simulink model "airbrakes"  (R2025b)
settings: Solver=VariableStepAuto  StartTime=0.0  StopTime=10.0  RelTol=1e-3
values from neighbouring files (symbols this model uses):
  baro_bias_initial = 1.0    (= 1)    [init_airbrake_model.m]
  baro_sigma_h = 0.5    [init_airbrake_model.m]
  burnout_time = motor_time(end)    [init_airbrake_model.m]
  Cd_body_bp = [0.45 0.45 0.43 0.42 0.44 0.50 0.65 0.75 0.62 0.52 0.48]    [init_airbrake_model.m]
  DeltaCd_ab_table = [ ... (first row only)    [init_airbrake_model.m]
  deploy_bp = [0 0.25 0.50 0.75 1.00]    [init_airbrake_model.m]
  deploy_rate_down = 6.67    [init_airbrake_model.m]
  deploy_rate_up = 6.67    [init_airbrake_model.m]
  g0 = 9.80665    [init_airbrake_model.m]
  imu_accel_range_g = 16    [init_airbrake_model.m]
  imu_bias_initial = 0.05    [init_airbrake_model.m]
  imu_delay = 0.005    [init_airbrake_model.m]
  imu_sigma_a = 0.15    [init_airbrake_model.m]
  Mach_ab_bp = Mach_bp    [init_airbrake_model.m]
  Mach_bp = [0 0.1 0.3 0.5 0.7 0.85 0.95 1.05 1.2 1.5 2.0]    [init_airbrake_model.m]
  mass_curve = linspace(m0, m_dry, numel(mass_time))    [init_airbrake_model.m]
  mass_time = motor_time    [init_airbrake_model.m]
  motor_thrust = [0 1200 2500 3300 3400 3200 2800 1900 700 100 0]    [init_airbrake_model.m]
  motor_time = [0 0.05 0.10 0.50 1.00 1.50 2.00 2.50 3.00 3.20 3.30]    [init_airbrake_model.m]
  Ts_baro = 0.02    [init_airbrake_model.m]
  Ts_imu = 0.005    [init_airbrake_model.m]
undefined symbols (not defined in the file or in its folder): bldc_tau
libraries: simulink x4
settings Model: Creator=parsa  LastModifiedBy=parsa

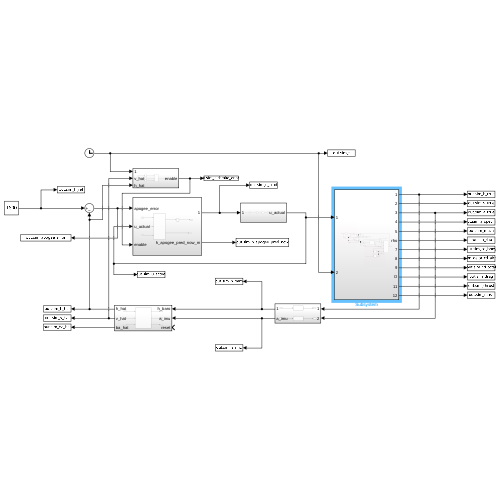
[thumbnail: Simulink's stored preview of the top-level diagram]
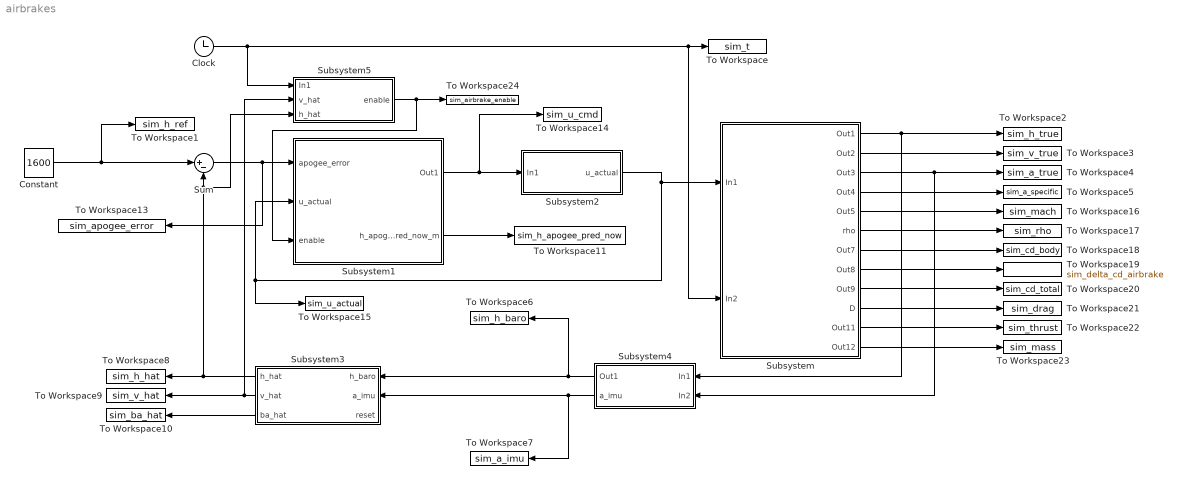
== system airbrakes ==
  Clock : Clock
  Constant : Constant  Value=1600
  Subsystem : Subsystem
  Subsystem1 : Subsystem
  Subsystem2 : Subsystem
  Subsystem3 : Subsystem
  Subsystem4 : Subsystem
  Subsystem5 : Subsystem
  Sum : Sum  Inputs=|+-
  To Workspace : ToWorkspace  VariableName=sim_t  SaveFormat=Timeseries  SampleTime=-1
  To Workspace1 : ToWorkspace  VariableName=sim_h_ref  SaveFormat=Timeseries  SampleTime=-1
  To Workspace10 : ToWorkspace  VariableName=sim_ba_hat  SaveFormat=Timeseries  SampleTime=-1
  To Workspace11 : ToWorkspace  VariableName=sim_h_apogee_pred_now  SaveFormat=Timeseries  SampleTime=-1
  To Workspace13 : ToWorkspace  VariableName=sim_apogee_error  SaveFormat=Timeseries  SampleTime=-1
  To Workspace14 : ToWorkspace  VariableName=sim_u_cmd  SaveFormat=Timeseries  SampleTime=-1
  To Workspace15 : ToWorkspace  VariableName=sim_u_actual  SaveFormat=Timeseries  SampleTime=-1
  To Workspace16 : ToWorkspace  VariableName=sim_mach  SaveFormat=Timeseries  SampleTime=-1
  To Workspace17 : ToWorkspace  VariableName=sim_rho  SaveFormat=Timeseries  SampleTime=-1
  To Workspace18 : ToWorkspace  VariableName=sim_cd_body  SaveFormat=Timeseries  SampleTime=-1
  To Workspace19 : ToWorkspace  VariableName=sim_delta_cd_airbrake  SaveFormat=Timeseries  SampleTime=-1
  To Workspace2 : ToWorkspace  VariableName=sim_h_true  SaveFormat=Timeseries  SampleTime=-1
  To Workspace20 : ToWorkspace  VariableName=sim_cd_total  SaveFormat=Timeseries  SampleTime=-1
  To Workspace21 : ToWorkspace  VariableName=sim_drag  SaveFormat=Timeseries  SampleTime=-1
  To Workspace22 : ToWorkspace  VariableName=sim_thrust  SaveFormat=Timeseries  SampleTime=-1
  To Workspace23 : ToWorkspace  VariableName=sim_mass  SaveFormat=Timeseries  SampleTime=-1
  To Workspace24 : ToWorkspace  VariableName=sim_airbrake_enable  SaveFormat=Timeseries  SampleTime=-1
  To Workspace3 : ToWorkspace  VariableName=sim_v_true  SaveFormat=Timeseries  SampleTime=-1
  To Workspace4 : ToWorkspace  VariableName=sim_a_true  SaveFormat=Timeseries  SampleTime=-1
  To Workspace5 : ToWorkspace  VariableName=sim_a_specific  SaveFormat=Timeseries  SampleTime=-1
  To Workspace6 : ToWorkspace  VariableName=sim_h_baro  SaveFormat=Timeseries  SampleTime=-1
  To Workspace7 : ToWorkspace  VariableName=sim_a_imu  SaveFormat=Timeseries  SampleTime=-1
  To Workspace8 : ToWorkspace  VariableName=sim_h_hat  SaveFormat=Timeseries  SampleTime=-1
  To Workspace9 : ToWorkspace  VariableName=sim_v_hat  SaveFormat=Timeseries  SampleTime=-1
  wires:
  Subsystem4/1(Out1) -> To Workspace6/1, Subsystem3/1(h_baro)
  Subsystem1/1(Out1) -> To Workspace14/1, Subsystem2/1(In1)
  Subsystem3/1(h_hat) -> Subsystem5/3(h_hat), Sum/2, To Workspace8/1
  Constant/1 -> To Workspace1/1, Sum/1
  Subsystem2/1(u_actual) -> To Workspace15/1, Subsystem1/2(u_actual), Subsystem/1(In1)
  Subsystem4/2(a_imu) -> To Workspace7/1, Subsystem3/2(a_imu)
  Clock/1 -> Subsystem5/1(In1), Subsystem/2(In2), To Workspace/1
  Subsystem3/2(v_hat) -> To Workspace9/1, Subsystem5/2(v_hat)
  Sum/1 -> To Workspace13/1, Subsystem1/1(apogee_error)
  Subsystem5/1(enable) -> To Workspace24/1, Subsystem1/3(enable)
  Subsystem3/3(ba_hat) -> To Workspace10/1
  Subsystem1/2(h_apogee_pred_now_m) -> To Workspace11/1
  Subsystem/1(Out1) -> Subsystem4/1(In1), To Workspace2/1
  Subsystem/2(Out2) -> To Workspace3/1
  Subsystem/3(Out3) -> Subsystem4/2(In2), To Workspace4/1
  Subsystem/4(Out4) -> To Workspace5/1
  Subsystem/5(Out5) -> To Workspace16/1
  Subsystem/6(rho) -> To Workspace17/1
  Subsystem/7(Out7) -> To Workspace18/1
  Subsystem/8(Out8) -> To Workspace19/1
  Subsystem/9(Out9) -> To Workspace20/1
  Subsystem/10(D) -> To Workspace21/1
  Subsystem/11(Out11) -> To Workspace22/1
  Subsystem/12(Out12) -> To Workspace23/1

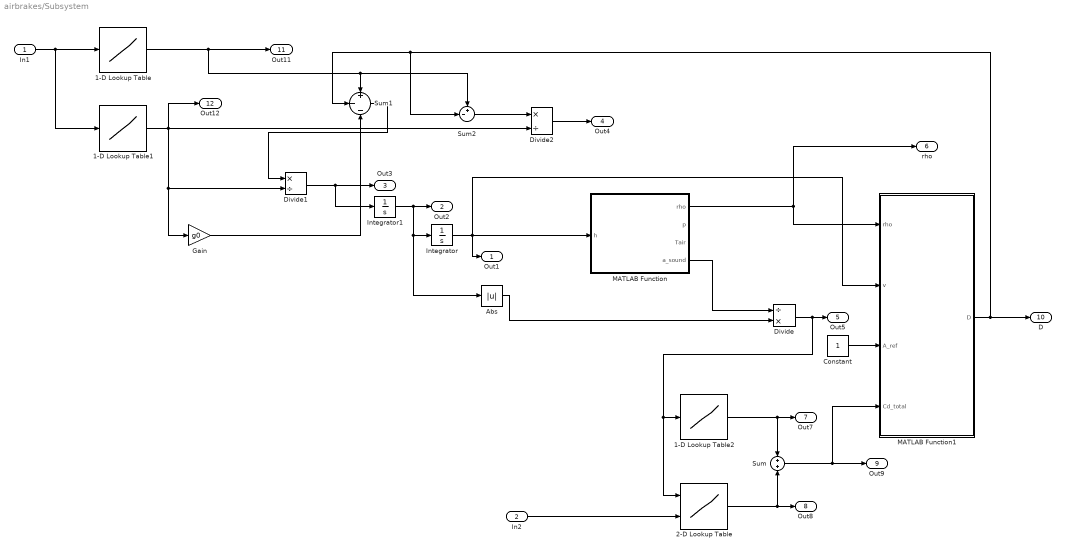
== system airbrakes/Subsystem ==
  In1 : Inport
  In2 : Inport  Port=2
  1-D Lookup Table : Lookup_n-D  NumberOfTableDimensions=1  BreakpointsForDimension1=motor_thrust  Table=motor_time  InternalRulePriority=Speed  RndMeth=Simplest
  1-D Lookup Table1 : Lookup_n-D  NumberOfTableDimensions=1  BreakpointsForDimension1=mass_time  Table=mass_curve  InternalRulePriority=Speed  RndMeth=Simplest
  1-D Lookup Table2 : Lookup_n-D  NumberOfTableDimensions=1  BreakpointsForDimension1=Mach_bp  Table=Cd_body_bp  InternalRulePriority=Speed  RndMeth=Simplest
  2-D Lookup Table : Lookup_n-D  BreakpointsForDimension1=deploy_bp  BreakpointsForDimension2=Mach_ab_bp  Table=DeltaCd_ab_table  InternalRulePriority=Speed  RndMeth=Simplest
      settings: InputPortMap=u0,u1
  Abs : Abs  SaturateOnIntegerOverflow=off
  Constant : Constant
  Divide : Product  Inputs=/*
  Divide1 : Product  Inputs=*/
  Divide2 : Product  Inputs=*/
  Gain : Gain  Gain=g0
  Integrator : Integrator
  Integrator1 : Integrator
  MATLAB Function : MATLAB Function  TreatAsAtomicUnit=on
  MATLAB Function1 : MATLAB Function  TreatAsAtomicUnit=on
  Sum : Sum  Inputs=+|+
  Sum1 : Sum  Inputs=+|-|-
  Sum2 : Sum  Inputs=+-|
  Out1 : Outport
  Out2 : Outport  Port=2
  Out3 : Outport  Port=3
  Out4 : Outport  Port=4
  Out5 : Outport  Port=5
  rho : Outport  Port=6
  Out7 : Outport  Port=7
  Out8 : Outport  Port=8
  Out9 : Outport  Port=9
  D : Outport  Port=10
  Out11 : Outport  Port=11
  Out12 : Outport  Port=12
  wires:
  In1/1 -> 1-D Lookup Table1/1, 1-D Lookup Table/1
  1-D Lookup Table/1 -> Sum2/1, Sum1/1, Out11/1
  1-D Lookup Table1/1 -> Out12/1, Divide2/2, Gain/1, Divide1/2
  Sum1/1 -> Divide1/1
  Divide1/1 -> Integrator1/1, Out3/1
  Integrator1/1 -> Out2/1, Abs/1, Integrator/1
  Integrator/1 -> Out1/1, MATLAB Function/1(h), MATLAB Function1/2(v)
  MATLAB Function/1(rho) -> MATLAB Function1/1(rho), rho/1
  MATLAB Function/4(a_sound) -> Divide/1
  Abs/1 -> Divide/2
  Divide/1 -> 2-D Lookup Table/1, 1-D Lookup Table2/1, Out5/1
  In2/1 -> 2-D Lookup Table/2
  1-D Lookup Table2/1 -> Out7/1, Sum/1
  2-D Lookup Table/1 -> Out8/1, Sum/2
  Sum/1 -> Out9/1, MATLAB Function1/4(Cd_total)
  Gain/1 -> Sum1/3
  MATLAB Function1/1(D) -> D/1, Sum2/2, Sum1/2
  Constant/1 -> MATLAB Function1/3(A_ref)
  Sum2/1 -> Divide2/1
  Divide2/1 -> Out4/1

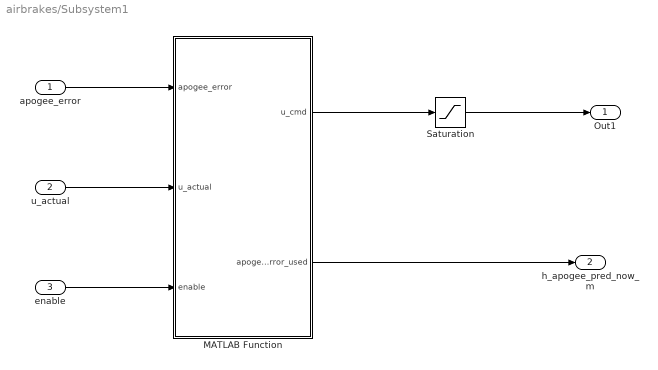
== system airbrakes/Subsystem1 ==
  apogee_error : Inport
  u_actual : Inport  Port=2
  enable : Inport  Port=3
  MATLAB Function : MATLAB Function  TreatAsAtomicUnit=on
  Saturation : Saturate  UpperLimit=1  LowerLimit=0
  Out1 : Outport
  h_apogee_pred_now_m : Outport  Port=2
  wires:
  MATLAB Function/1(u_cmd) -> Saturation/1
  Saturation/1 -> Out1/1
  MATLAB Function/2(apogee_error_used) -> h_apogee_pred_now_m/1
  enable/1 -> MATLAB Function/3(enable)
  u_actual/1 -> MATLAB Function/2(u_actual)
  apogee_error/1 -> MATLAB Function/1(apogee_error)

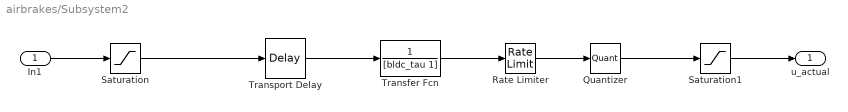
== system airbrakes/Subsystem2 ==
  In1 : Inport
  Quantizer : Quantizer  QuantizationInterval=bldc_quant_step
  Rate Limiter : RateLimiter  RisingSlewLimit=deploy_rate_up  FallingSlewLimit=-deploy_rate_down  SampleTimeMode=inherited
  Saturation : Saturate  UpperLimit=1  LowerLimit=0
  Saturation1 : Saturate  UpperLimit=1  LowerLimit=0
  Transfer Fcn : TransferFcn  Denominator=[bldc_tau 1]
  Transport Delay : TransportDelay
  u_actual : Outport
  wires:
  In1/1 -> Saturation/1
  Saturation/1 -> Transport Delay/1
  Transport Delay/1 -> Transfer Fcn/1
  Transfer Fcn/1 -> Rate Limiter/1
  Rate Limiter/1 -> Quantizer/1
  Quantizer/1 -> Saturation1/1
  Saturation1/1 -> u_actual/1

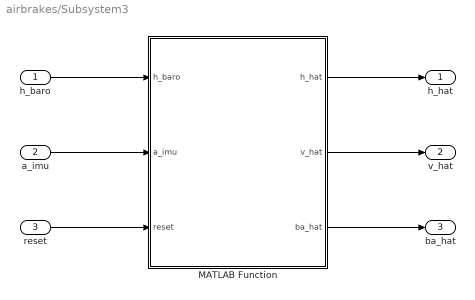
== system airbrakes/Subsystem3 ==
  h_baro : Inport
  a_imu : Inport  Port=2
  reset : Inport  Port=3
  MATLAB Function : MATLAB Function  TreatAsAtomicUnit=on
  h_hat : Outport
  v_hat : Outport  Port=2
  ba_hat : Outport  Port=3
  wires:
  reset/1 -> MATLAB Function/3(reset)
  a_imu/1 -> MATLAB Function/2(a_imu)
  h_baro/1 -> MATLAB Function/1(h_baro)
  MATLAB Function/1(h_hat) -> h_hat/1
  MATLAB Function/2(v_hat) -> v_hat/1
  MATLAB Function/3(ba_hat) -> ba_hat/1

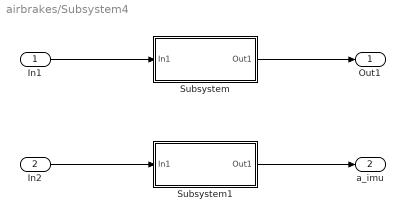
== system airbrakes/Subsystem4 ==
  In1 : Inport
  In2 : Inport  Port=2
  Subsystem : Subsystem
  Subsystem1 : Subsystem
  Out1 : Outport
  a_imu : Outport  Port=2
  wires:
  In2/1 -> Subsystem1/1(In1)
  Subsystem1/1(Out1) -> a_imu/1
  Subsystem/1(Out1) -> Out1/1
  In1/1 -> Subsystem/1(In1)

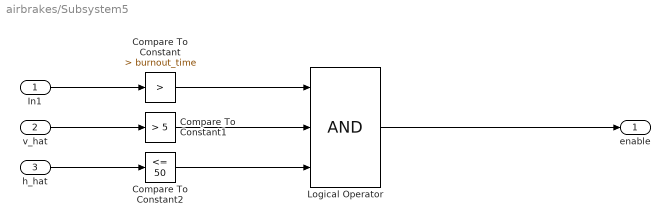
== system airbrakes/Subsystem5 ==
  In1 : Inport
  v_hat : Inport  Port=2
  h_hat : Inport  Port=3
  Compare To Constant : simulink/Logic and Bit Operations/Compare To Constant  relop=>  const=burnout_time  OutDataTypeStr=boolean
  Compare To Constant1 : simulink/Logic and Bit Operations/Compare To Constant  relop=>  const=5  OutDataTypeStr=boolean
  Compare To Constant2 : simulink/Logic and Bit Operations/Compare To Constant  relop=<=  const=50  OutDataTypeStr=boolean
  Logical Operator : Logic  Inputs=3  AllPortsSameDT=off  OutDataTypeStr=boolean
  enable : Outport
  wires:
  In1/1 -> Compare To Constant/1
  Compare To Constant/1 -> Logical Operator/1
  v_hat/1 -> Compare To Constant1/1
  h_hat/1 -> Compare To Constant2/1
  Compare To Constant1/1 -> Logical Operator/2
  Compare To Constant2/1 -> Logical Operator/3
  Logical Operator/1 -> enable/1

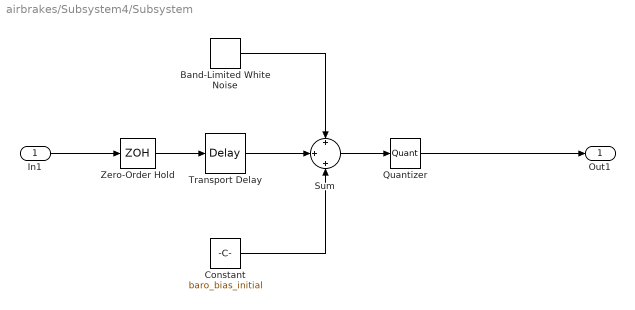
== system airbrakes/Subsystem4/Subsystem ==
  In1 : Inport
  Band-Limited White Noise : simulink/Sources/Band-Limited White Noise  Cov=[baro_sigma_h^2 * Ts_baro]  Ts=Ts_baro  seed=[23341]
  Constant : Constant  Value=baro_bias_initial
  Quantizer : Quantizer
  Sum : Sum  Inputs=+|+|+
  Transport Delay : TransportDelay
  Zero-Order Hold : ZeroOrderHold  SampleTime=-1
  Out1 : Outport
  wires:
  In1/1 -> Zero-Order Hold/1
  Zero-Order Hold/1 -> Transport Delay/1
  Band-Limited White Noise/1 -> Sum/1
  Transport Delay/1 -> Sum/2
  Constant/1 -> Sum/3
  Sum/1 -> Quantizer/1
  Quantizer/1 -> Out1/1

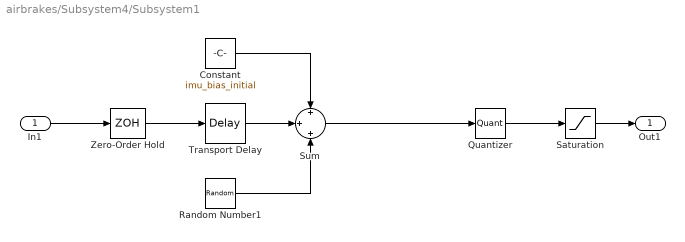
== system airbrakes/Subsystem4/Subsystem1 ==
  In1 : Inport
  Constant : Constant  Value=imu_bias_initial
  Quantizer : Quantizer  QuantizationInterval=imu_quant_step
  Random Number1 : RandomNumber  Variance=imu_sigma_a^2  SampleTime=Ts_imu
  Saturation : Saturate  UpperLimit=imu_accel_range_g*g0  LowerLimit=-imu_accel_range_g*g0
  Sum : Sum  Inputs=+|+|+
  Transport Delay : TransportDelay  DelayTime=imu_delay
  Zero-Order Hold : ZeroOrderHold  SampleTime=Ts_imu
  Out1 : Outport
  wires:
  In1/1 -> Zero-Order Hold/1
  Saturation/1 -> Out1/1
  Quantizer/1 -> Saturation/1
  Constant/1 -> Sum/1
  Zero-Order Hold/1 -> Transport Delay/1
  Random Number1/1 -> Sum/3
  Sum/1 -> Quantizer/1
  Transport Delay/1 -> Sum/2

== matlab function airbrakes/Subsystem/MATLAB Function1 ==
  data: rho input; D output; v input; A_ref input; Cd_total input
function D = drag_force(rho, v, A_ref, Cd_total)
%#codegen
D = 0.5 * rho * v * abs(v) * A_ref * Cd_total;

== matlab function airbrakes/Subsystem/MATLAB Function ==
  data: h input; rho output; p output; Tair output; a_sound output
function [rho, p, Tair, a_sound] = atmosphere_model(h)
%#codegen

g0 = 9.80665;
rho0 = 1.225;
T0 = 288.15;
p0 = 101325;
L = 0.0065;
R_air = 287.05;
gamma_air = 1.4;

if h < 0
    h = 0;
end

Tair = T0 - L*h;

if Tair < 216.65
    Tair = 216.65;
end

p = p0 * (Tair/T0)^(g0/(R_air*L));
rho = p/(R_air*Tair);
a_sound = sqrt(gamma_air*R_air*Tair);

== matlab function airbrakes/Subsystem3/MATLAB Function ==
  data: h_baro input; h_hat output; a_imu input; reset input; v_hat output; ba_hat output
function [h_hat, v_hat, ba_hat] = altitude_velocity_kf(h_baro, a_imu, reset)
%#codegen

Ts = 0.05;
g0 = 9.80665;

Q = diag([0.01^2, 0.1^2, 0.03^2]);
R = 0.5^2;

persistent x P initialized

if isempty(initialized) || reset
    x = [h_baro; 0; 0.05];
    P = diag([10^2, 10^2, 0.5^2]);
    initialized = true;
end

h = x(1);
v = x(2);
ba = x(3);

a_corr = a_imu - ba - g0;

x_pred = [
    h + v*Ts + 0.5*a_corr*Ts^2;
    v + a_corr*Ts;
    ba
];

F = [
    1, Ts, -0.5*Ts^2;
    0,  1, -Ts;
    0,  0,  1
];

P_pred = F*P*F' + Q;

H = [1 0 0];

y = h_baro - H*x_pred;
S = H*P_pred*H' + R;
K = P_pred*H'/S;

x = x_pred + K*y;
P = (eye(3) - K*H)*P_pred;

h_hat = x(1);
v_hat = x(2);
ba_hat = x(3);

== matlab function airbrakes/Subsystem1/MATLAB Function ==
  data: apogee_error input; u_cmd output; u_actual input; enable input; apogee_error_used output
function [u_cmd, apogee_error_used] = fakeshi(apogee_error, u_actual, enable)
%#codegen

if enable == 0
    u_cmd = 0;
    apogee_error_used = apogee_error;
    return;
end

deadband_m = 5;
Kp = 1/300;

u_min = 0;
u_max = 1;

apogee_error_used = apogee_error;

if abs(apogee_error) <= deadband_m
    u_cmd = u_actual;
    return;
end

if apogee_error > 0
    u_cmd = Kp * apogee_error;
else
    u_cmd = 0;
end

if u_cmd > u_max
    u_cmd = u_max;
elseif u_cmd < u_min
    u_cmd = u_min;
end

end
